simulink model "cvoo_g19_init"  (R2020a)
settings: Solver=VariableStepAuto  StartTime=0.0  StopTime=10.0  RelTol=1e-3
values from neighbouring files (symbols this model uses):
  a_h = [ ... (first row only)    [main.m]    (also in main_controlo_altitude.m; main_novo.m; main_thomas.m; main_thomas_rp1.m)
  b_h_sf = b_h(:,[1,3])    [main.m]    (also in main_controlo_altitude.m; main_novo.m)
  c_h = eye(size(a_h))    [main.m]    (also in main_controlo_altitude.m; main_novo.m; main_thomas.m; main_thomas_rp1.m)
  d_h_sf = d_h(:,[1,3])    [main.m]    (also in main_controlo_altitude.m; main_novo.m)
  K_lqr = lqr(a_h_pt_int, b_h_pt_int, Q, R)    [Ponto3.m]    (also in main.m = lqr(a_h_SAE, b_h_sf, Q, R); main_controlo_altitude.m = lqr(a_h_int, b_h_sf_int, Q, R); main_novo.m)
  x0 = [0 0 0 0]    [Ponto3.m]    (also in main.m = [0 0 0 0 0]; main_controlo_altitude.m; main_novo.m)
settings Model: Creator=josem  LastModifiedBy=josem

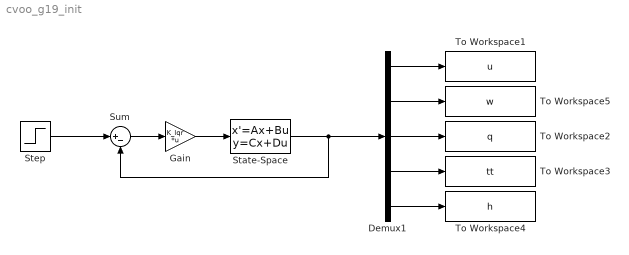
== system cvoo_g19_init ==
  Demux1 : Demux  Outputs=5
  Gain : Gain  Gain=K_lqr  Multiplication=Matrix(K*u)
  State-Space : StateSpace  A=a_h  B=b_h_sf  C=c_h  D=d_h_sf  InitialCondition=x0
  Step : Step  Before=x0'  After=reference'  SampleTime=0  VectorParams1D=off
  Sum : Sum  Inputs=|+-
  To Workspace1 : ToWorkspace  VariableName=u  SampleTime=-1
  To Workspace2 : ToWorkspace  VariableName=q  SampleTime=-1
  To Workspace3 : ToWorkspace  VariableName=tt  SampleTime=-1
  To Workspace4 : ToWorkspace  VariableName=h  SampleTime=-1
  To Workspace5 : ToWorkspace  VariableName=w  SampleTime=-1
  wires:
  State-Space/1 -> Sum/2, Demux1/1
  Demux1/2 -> To Workspace5/1
  Demux1/1 -> To Workspace1/1
  Demux1/3 -> To Workspace2/1
  Demux1/4 -> To Workspace3/1
  Demux1/5 -> To Workspace4/1
  Gain/1 -> State-Space/1
  Sum/1 -> Gain/1
  Step/1 -> Sum/1
